simulink model "Three_Phase_inverter"  (R2023b)
settings: Solver=VariableStepDiscrete  StartTime=0.0  StopTime=1  RelTol=1e-3
libraries: spsVoltageMeasurementLib x7, spsIGBTLib x6, spsSeriesRLCBranchLib x6, spsCurrentMeasurementLib x3, spsDCVoltageSourceLib x1, simulink x1, sps_lib x1
settings Model: Creator=prade  LastModifiedBy=prade
settings DataIOCC: SaveFormat=StructureWithTime  SignalLoggingName=Three_Phaseinverter
settings SimscapeCC: SimscapeLogType=all  SimscapeLogName=Three_Phaseinverter  SimscapeLogLimitData=off

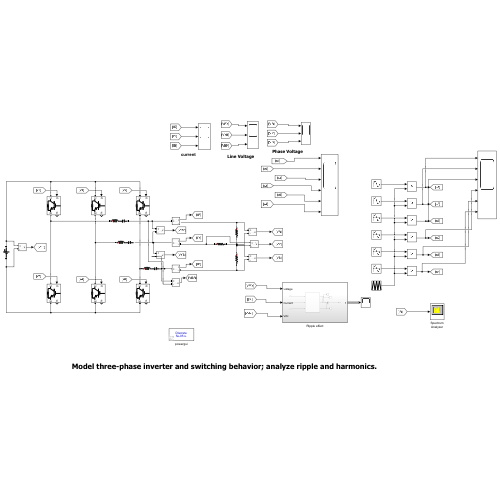
[thumbnail: Simulink's stored preview of the top-level diagram]
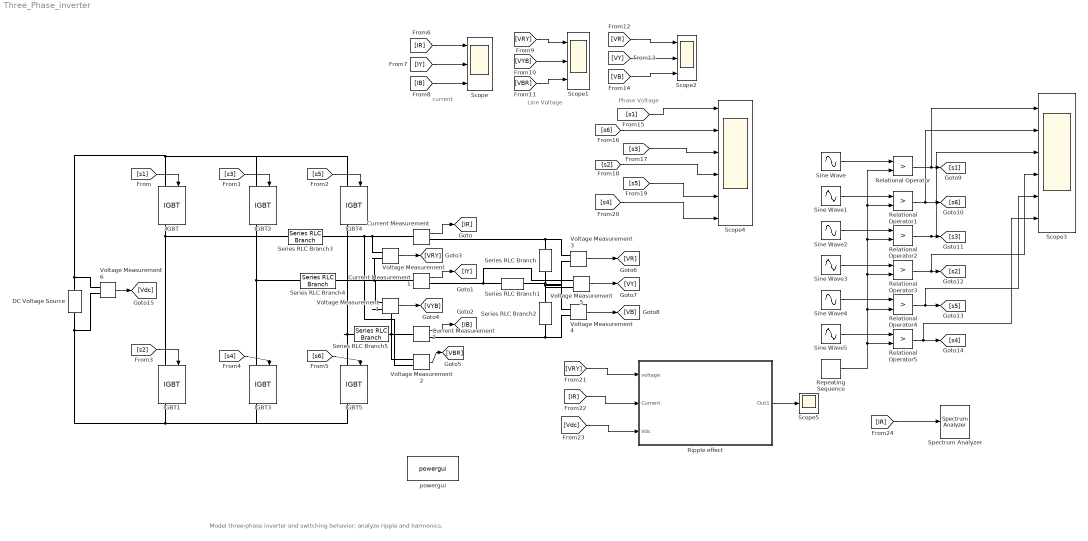
== system Three_Phase_inverter ==
  note: Model three-phase inverter and switching behavior; analyze ripple and harmonics.
  note: Phase Voltage
  note: Line Voltage
  note: current
  Current Measurement : spsCurrentMeasurementLib/Current Measurement  PhasorSimulation=off  OutputType=Complex  PSBequivalent=0
  Current Measurement1 : spsCurrentMeasurementLib/Current Measurement  PhasorSimulation=off  OutputType=Complex  PSBequivalent=0
  Current Measurement2 : spsCurrentMeasurementLib/Current Measurement  PhasorSimulation=off  OutputType=Complex  PSBequivalent=0
  DC Voltage Source : spsDCVoltageSourceLib/DC Voltage Source  Amplitude=100  Measurements=None
  IGBT{,1..5} (6 alike) : spsIGBTLib/IGBT  Ron=0.001  Lon=0  Vf=1  Tf=1e-6  Tt=2e-6  IC=0  Rs=1e5  Cs=inf  Measurements=on
  Relational Operator{,1..5} (6 alike) : RelationalOperator  Operator=>  OutDataTypeStr=boolean  RndMeth=Simplest  InputSameDT=off
  Repeating Sequence : simulink/Sources/Repeating Sequence  rep_seq_t=[0 0.02/40 0.02/20]  rep_seq_y=[0 2 0]
  Ripple effect : Subsystem
  Scope : Scope  NumInputPorts=3
  Scope1 : Scope  NumInputPorts=3
  Scope2 : Scope  NumInputPorts=3
  Scope3 : Scope  NumInputPorts=6
  Scope4 : Scope  NumInputPorts=6
  Scope5 : Scope
  Series RLC Branch : spsSeriesRLCBranchLib/Series RLC Branch  LConnTagsString=__new0  RConnTagsString=__new0  BranchType=R  Resistance=1  Inductance=1e-3  SetiL0=off  InitialCurrent=0  Capacitance=1e-6  Setx0=off  InitialVoltage=0  Measurements=None
  Series RLC Branch1 : spsSeriesRLCBranchLib/Series RLC Branch  LConnTagsString=__new0  RConnTagsString=__new0  BranchType=R  Resistance=1  Inductance=1e-3  SetiL0=off  InitialCurrent=0  Capacitance=1e-6  Setx0=off  InitialVoltage=0  Measurements=None
  Series RLC Branch2 : spsSeriesRLCBranchLib/Series RLC Branch  LConnTagsString=__new0  RConnTagsString=__new0  BranchType=R  Resistance=1  Inductance=1e-3  SetiL0=off  InitialCurrent=0  Capacitance=1e-6  Setx0=off  InitialVoltage=0  Measurements=None
  Series RLC Branch3 : spsSeriesRLCBranchLib/Series RLC Branch  LConnTagsString=__new0  RConnTagsString=__new0  BranchType=LC  Resistance=1  Inductance=1e-3  SetiL0=off  InitialCurrent=0  Capacitance=1e-6  Setx0=off  InitialVoltage=0  Measurements=None
  Series RLC Branch4 : spsSeriesRLCBranchLib/Series RLC Branch  LConnTagsString=__new0  RConnTagsString=__new0  BranchType=LC  Resistance=1  Inductance=1e-3  SetiL0=off  InitialCurrent=0  Capacitance=1e-6  Setx0=off  InitialVoltage=0  Measurements=None
  Series RLC Branch5 : spsSeriesRLCBranchLib/Series RLC Branch  LConnTagsString=__new0  RConnTagsString=__new0  BranchType=LC  Resistance=1  Inductance=1e-3  SetiL0=off  InitialCurrent=0  Capacitance=1e-6  Setx0=off  InitialVoltage=0  Measurements=None
  Sine Wave : Sin  Frequency=2*pi*50  SampleTime=0
  Sine Wave1 : Sin  Frequency=2*pi*50  Phase=60*(pi/180)  SampleTime=0
  Sine Wave2 : Sin  Frequency=2*pi*50  Phase=120*(pi/180)  SampleTime=0
  Sine Wave3 : Sin  Frequency=2*pi*50  Phase=180*(pi/180)  SampleTime=0
  Sine Wave4 : Sin  Frequency=2*pi*50  Phase=240*(pi/180)  SampleTime=0
  Sine Wave5 : Sin  Frequency=2*pi*50  Phase=300*(pi/180)  SampleTime=0
  Spectrum Analyzer : SpectrumAnalyzer  WindowPosition=[283.000000,134.000000,800.000000,500.000000,]  ScopeFrameLocation=window  Method=Welch  PlotAsTwoSidedSpectrum=off  AveragingMethod=Exponential  YLimits=[-64.30571468,9.30366777]  SelectedToolstripTab=spectrumAnalyzerToolstrip.spectrumTab
  Voltage Measurement{,1..6} (7 alike) : spsVoltageMeasurementLib/Voltage Measurement  PhasorSimulation=off  OutputType=Complex  PSBequivalent=0
  powergui : sps_lib/powergui  Priority=1  SimulationMode=Discrete  SampleTime=50e-6  frequency=60  Iterations=50  frequencyindice=0  Pbase=100e6  ErrMax=1e-4  UnitsV=kV  UnitsW=MW  buscounter=0  FunctionMessages=off  echomessages=off  EnableUseOfTLC=off  CurrentSourceSwitches=off  DisableSnubberDevices=off  DisableRonSwitches=off  DisableVfSwitches=off  DisplayEquations=off  AutomaticDiscreteSolvers=off  SolverType=Tustin/Backward Euler (TBE)  Interpol=off  ExternalGateDelay=off  methode=off  Ts=100  x0status=blocks  SPID=on  SwTol=0  HookPort=off  NonlinearTolerance=1e-4  nMaxIteration=100  ContinueOnMaxIteration=off  RestoreLinks=warning  ResistiveCurrentMeasurement=off  Frange=[0:2:500]  Ylog=off  Xlog=on  ShowGrid=off  save=off  variable=ZData  structure=0  ZoomFFT=off  StartTime=0.0  cycles=1  DisplayStyle=1  fundamental=60  FreqAxis=off  MaxFrequency=1000  frequencyindicesteady=1  RmsSteady=1  display=off
  wires:
  [s1] -> IGBT/1
  [s3] -> IGBT2/1
  [s5] -> IGBT4/1
  [s2] -> IGBT1/1
  [s4] -> IGBT3/1
  [s6] -> IGBT5/1
  Current Measurement/1 -> [IR]
  Current Measurement1/1 -> [IY]
  Current Measurement2/1 -> [IB]
  Voltage Measurement/1 -> [VRY]
  Voltage Measurement1/1 -> [VYB]
  Voltage Measurement2/1 -> [VBR]
  Voltage Measurement3/1 -> [VR]
  Voltage Measurement5/1 -> [VY]
  Voltage Measurement4/1 -> [VB]
  [IR] -> Scope/1
  [IY] -> Scope/2
  [IB] -> Scope/3
  [VRY] -> Scope1/1
  [VYB] -> Scope1/2
  [VBR] -> Scope1/3
  [VR] -> Scope2/1
  [VY] -> Scope2/2
  [VB] -> Scope2/3
  Sine Wave/1 -> Relational Operator/1
  Sine Wave1/1 -> Relational Operator1/1
  Sine Wave2/1 -> Relational Operator2/1
  Sine Wave3/1 -> Relational Operator3/1
  Sine Wave4/1 -> Relational Operator4/1
  Sine Wave5/1 -> Relational Operator5/1
  Repeating Sequence/1 -> Relational Operator5/2, Relational Operator4/2, Relational Operator3/2, Relational Operator2/2, Relational Operator1/2, Relational Operator/2
  Relational Operator/1 -> Scope3/1, [s1]
  Relational Operator1/1 -> Scope3/2, [s6]
  Relational Operator2/1 -> Scope3/3, [s3]
  Relational Operator3/1 -> Scope3/4, [s2]
  Relational Operator4/1 -> Scope3/5, [s5]
  Relational Operator5/1 -> Scope3/6, [s4]
  [s1] -> Scope4/1
  [s6] -> Scope4/2
  [s3] -> Scope4/3
  [s2] -> Scope4/4
  [s4] -> Scope4/6
  [s5] -> Scope4/5
  [VRY] -> Ripple effect/1(voltage)
  [IR] -> Ripple effect/2(Current)
  Voltage Measurement6/1 -> [Vdc]
  [Vdc] -> Ripple effect/3(Vdc)
  Ripple effect/1(Out1) -> Scope5/1
  [IR] -> Spectrum Analyzer/1
  connections:
  DC Voltage Source/RConn1 -- Voltage Measurement6/LConn1 -- IGBT2/LConn1 -- IGBT4/LConn1 -- IGBT/LConn1
  IGBT1/LConn1 -- Series RLC Branch3/LConn1 -- IGBT/RConn1
  IGBT3/LConn1 -- Series RLC Branch4/LConn1 -- IGBT2/RConn1
  IGBT4/RConn1 -- Series RLC Branch5/LConn1 -- IGBT5/LConn1
  DC Voltage Source/LConn1 -- Voltage Measurement6/LConn2 -- IGBT5/RConn1 -- IGBT3/RConn1 -- IGBT1/RConn1
  Series RLC Branch1/LConn1 -- Voltage Measurement5/LConn1 -- Current Measurement1/RConn1
  Series RLC Branch/RConn1 -- Voltage Measurement5/LConn2 -- Series RLC Branch2/LConn1 -- Voltage Measurement4/LConn1 -- Voltage Measurement3/LConn2 -- Series RLC Branch1/RConn1
  Current Measurement/RConn1 -- Voltage Measurement3/LConn1 -- Series RLC Branch/LConn1
  Series RLC Branch2/RConn1 -- Voltage Measurement4/LConn2 -- Current Measurement2/RConn1
  Voltage Measurement/LConn1 -- Series RLC Branch3/RConn1 -- Voltage Measurement2/LConn2 -- Current Measurement/LConn1
  Voltage Measurement1/LConn1 -- Series RLC Branch4/RConn1 -- Voltage Measurement/LConn2 -- Current Measurement1/LConn1
  Voltage Measurement1/LConn2 -- Current Measurement2/LConn1 -- Series RLC Branch5/RConn1 -- Voltage Measurement2/LConn1

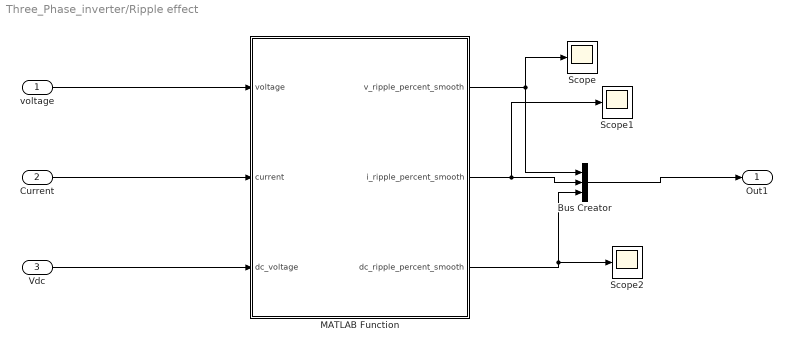
== system Three_Phase_inverter/Ripple effect ==
  voltage : Inport
  Current : Inport  Port=2
  Vdc : Inport  Port=3
  Bus Creator : BusCreator  Inputs=3
  MATLAB Function : MATLAB Function  TreatAsAtomicUnit=on
  Scope : Scope
  Scope1 : Scope
  Scope2 : Scope
  Out1 : Outport
  wires:
  voltage/1 -> MATLAB Function/1(voltage)
  Current/1 -> MATLAB Function/2(current)
  Vdc/1 -> MATLAB Function/3(dc_voltage)
  MATLAB Function/1(v_ripple_percent_smooth) -> Bus Creator/1, Scope/1
  MATLAB Function/2(i_ripple_percent_smooth) -> Scope1/1, Bus Creator/2
  MATLAB Function/3(dc_ripple_percent_smooth) -> Scope2/1, Bus Creator/3
  Bus Creator/1 -> Out1/1

== matlab function Three_Phase_inverter/Ripple effect/MATLAB Function ==
  data: voltage input; v_ripple_percent_smooth output; current input; dc_voltage input; i_ripple_percent_smooth output; dc_ripple_percent_smooth output
function [v_ripple_percent_smooth, i_ripple_percent_smooth, dc_ripple_percent_smooth] = improved_ripple_calc(voltage, current, dc_voltage)
%#codegen

% Improved ripple calculation with smoothing and better filtering

persistent v_buffer i_buffer dc_buffer buffer_idx N;
persistent v_ripple_history i_ripple_history dc_ripple_history;
persistent history_idx history_size initialized;

% Initialize on first call
if isempty(initialized)
    N = 400;  % Larger buffer for better frequency resolution
    history_size = 50;  % Smoothing window
    
    % Signal buffers
    v_buffer = zeros(N, 1);
    i_buffer = zeros(N, 1);  
    dc_buffer = zeros(N, 1);
    buffer_idx = 1;
    
    % Ripple history for smoothing
    v_ripple_history = zeros(history_size, 1);
    i_ripple_history = zeros(history_size, 1);
    dc_ripple_history = zeros(history_size, 1);
    history_idx = 1;
    
    initialized = true;
    
    % Return zero initially
    v_ripple_percent_smooth = 0;
    i_ripple_percent_smooth = 0;
    dc_ripple_percent_smooth = 0;
    return;
end

% Store current values in circular buffer
v_buffer(buffer_idx) = voltage;
i_buffer(buffer_idx) = current;
dc_buffer(buffer_idx) = dc_voltage;

% Calculate ripple only when buffer has enough samples
if buffer_idx >= N/2  % At least half buffer filled
    
    %% Advanced Voltage Ripple Analysis
    % Remove DC component
    v_mean = mean(v_buffer(1:min(buffer_idx, N)));
    v_centered = v_buffer(1:min(buffer_idx, N)) - v_mean;
    
    % Calculate RMS of AC components
    v_ac_rms = sqrt(mean(v_centered.^2));
    
    % Estimate fundamental component (50Hz)
    % Simple approach: fit sine wave to remove fundamental
    n_samples = min(buffer_idx, N);
    t_samples = (0:n_samples-1)';
    
    % Approximate fundamental removal
    fundamental_est = fit_fundamental(v_centered, 50, 10000);  % 50Hz, 10kHz sampling
    v_ripple_component = v_centered - fundamental_est;
    
    % Calculate ripple RMS
    v_ripple_rms = sqrt(mean(v_ripple_component.^2));
    
    % Ripple factor as percentage of fundamental
    v_fundamental_rms = sqrt(mean(fundamental_est.^2));
    if v_fundamental_rms > 1e-3
        v_ripple_current = (v_ripple_rms / v_fundamental_rms) * 100;
    else
        v_ripple_current = (v_ripple_rms / abs(v_mean)) * 100;
    end
    
    %% Current Ripple Analysis (similar approach)
    i_mean = mean(i_buffer(1:min(buffer_idx, N)));
    i_centered = i_buffer(1:min(buffer_idx, N)) - i_mean;
    
    i_fundamental_est = fit_fundamental(i_centered, 50, 10000);
    i_ripple_component = i_centered - i_fundamental_est;
    i_ripple_rms = sqrt(mean(i_ripple_component.^2));
    
    i_fundamental_rms = sqrt(mean(i_fundamental_est.^2));
    if i_fundamental_rms > 1e-3
        i_ripple_current = (i_ripple_rms / i_fundamental_rms) * 100;
    else
        i_ripple_current = (i_ripple_rms / abs(i_mean)) * 100;
    end
    
    %% DC Ripple Analysis
    dc_samples = dc_buffer(1:min(buffer_idx, N));
    dc_mean = mean(dc_samples);
    dc_max = max(dc_samples);
    dc_min = min(dc_samples);
    
    if dc_mean > 1
        dc_ripple_current = ((dc_max - dc_min) / (2 * dc_mean)) * 100;
    else
        dc_ripple_current = 0;
    end
    
    %% Store in smoothing history
    v_ripple_history(history_idx) = min(v_ripple_current, 50);  % Clamp extreme values
    i_ripple_history(history_idx) = min(i_ripple_current, 100);
    dc_ripple_history(history_idx) = min(dc_ripple_current, 20);
    
    %% Apply smoothing (moving average)
    valid_history = min(history_idx, history_size);
    v_ripple_percent_smooth = mean(v_ripple_history(1:valid_history));
    i_ripple_percent_smooth = mean(i_ripple_history(1:valid_history));
    dc_ripple_percent_smooth = mean(dc_ripple_history(1:valid_history));
    
    % Update history index
    history_idx = history_idx + 1;
    if history_idx > history_size
        history_idx = 1;
    end
    
else
    % Not enough samples - return previous smoothed values
    if history_idx > 1
        v_ripple_percent_smooth = mean(v_ripple_history(1:min(history_idx-1, history_size)));
        i_ripple_percent_smooth = mean(i_ripple_history(1:min(history_idx-1, history_size)));
        dc_ripple_percent_smooth = mean(dc_ripple_history(1:min(history_idx-1, history_size)));
    else
        v_ripple_percent_smooth = 0;
        i_ripple_percent_smooth = 0;
        dc_ripple_percent_smooth = 0;
    end
end

% Update buffer index
buffer_idx = buffer_idx + 1;
if buffer_idx > N
    buffer_idx = 1;
end

end

%% Helper function to estimate and remove fundamental component
function fundamental_component = fit_fundamental(signal, freq, fs)
    n_samples = length(signal);
    t = (0:n_samples-1)' / fs;
    
    % Simple DFT-based fundamental estimation
    omega = 2 * pi * freq;
    
    % Calculate coefficients for fundamental sine and cosine
    cos_coeff = (2/n_samples) * sum(signal .* cos(omega * t));
    sin_coeff = (2/n_samples) * sum(signal .* sin(omega * t));
    
    % Reconstruct fundamental
    fundamental_component = cos_coeff * cos(omega * t) + sin_coeff * sin(omega * t);
end
